simulink model "RM3_copy"  (R2017b)
settings: Solver=ode4  StartTime=0  StopTime=14400  FixedStep=0.1  MaxStep=0.1  RelTol=1e-3  EnableMultiTasking=on
values from neighbouring files (symbols this model uses):
  m = min(Out,[],2)    [ContinousControl.m]    (also in RL.m; RealTime_modif22.m)
  N = No*n    (= 60)    [ACTOR_CRITIC & SARSA.m]    (also in TDlearningExampleEforPosting.m)
  s = tf('s')    [Fe_extract.m]    (also in InputDataExtraction.m; LetsStartIt.m; SafeLetsStartIt.m; StateExtraction.m)
  states_space = states_spaceP    [ContinousControl.m]    (also in Forward_step.m = states_spaceP([1:9 6*9+1:9*7 15*9+1:9*16 5*9+1:9*6],:); RealTime_modif22.m)
  X = YX(:,2:end)    [L2adaptivepredictor.m]
  Y = YX(:,1)    [L2adaptivepredictor.m]
undefined symbols (not defined in the file or in its folder): body, constraint, pto, Z
libraries: nesl_utility x8, sm_lib x5, WECSim_Lib x4
settings Model: Creator=mlawson  LastModifiedBy=ghleila
settings SolverCC: ZeroCrossControl=DisableAll  AlgebraicLoopSolver=LineSearch  AutoInsertRateTranBlk=on
settings DataIOCC: SaveFormat=Array  SaveOutput=off  SaveTime=off
settings OptimizationCC: LifeSpan=inf  SimCompilerOptimization=on
settings DebuggingCC: UnderspecifiedInitializationDetection=Classic  MergeDetectMultiDrivingBlocksExec=none  SolverPrmCheckMsg=warning  AllowSymbolicDim=off  StateNameClashWarn=warning  SFUnexpectedBacktrackingDiag=warning  SFNoUnconditionalDefaultTransitionDiag=warning  SFExecutionAtInitializationDiag=none
settings HardwareCC: ProdBitPerPointer=32  ProdBitPerSizeT=32  ProdBitPerPtrDiffT=32  ProdLargestAtomicFloat=None  ProdIntDivRoundTo=Undefined  ProdEndianess=Unspecified  ProdWordSize=32  ProdHWDeviceType=32-bit Generic
settings ModelReferenceCC: PropagateSignalLabelsOutOfModel=off
settings CodeAppCC: StateflowObjectComments=on
settings GRTTargetCC: TargetLangStandard=C89/C90 (ANSI)  GeneratePreprocessorConditionals=Disable all
settings ConfigComp: CovMetricSettings=dw  CovHtmlReporting=on  CovSaveCumulativeToWorkspaceVar=on  CovSaveSingleToWorkspaceVar=on  CovExternalEMLEnable=off  CovSFcnEnable=off
settings SimscapeCC: SimscapeNormalizeSystem=off
settings ConfigurationSet: Description=SimMechanics 2G
settings ExplorerConfigSet: InternalSimMechanicsExplorerSettings="<ExplorerConfiguration><canonicalview>default</canonicalview><TilePanel><TileInfo><Tiles Columns=\"1\" Count=\"1\" Rows=\"1\"><Column Left=\"2\" Weight=\"1\"/><Column Left=\"1335\"/><Row Top=\"2\" Weight=\"1\"/><Row Top=\"911\"/><Tile Height=\"1\" Width=\"1\" X=\"0\" Y=\"0\"/></Tiles></TileInfo><SceneInfo><SceneViewer><BGColor><R>0.60000002384185791</R><G>0.60000002384185791</G><B>0.60000002384185791</B></BGColor><Camera><Position><X>365.37645888990272</X><Y>-369.82486814446582</Y><Z>359.64809521743916</Z></Position><Center><X>-6.7351450971904585</X><Y>2.2867358426280204</Y><Z>-12.463508769654169</Z></Center><Up><X>-0.40824829046386307</X><Y>0.40824829046386307</Y><Z>0.81649658092772615</Z></Up><Left>-57.820127362122818</Left><Right>57.820127362122818</Right><Bottom>-38.308817187253304</Bottom><Top>38.308817187253304</Top></Camera></SceneViewer></SceneInfo></TilePanel></ExplorerConfiguration>"

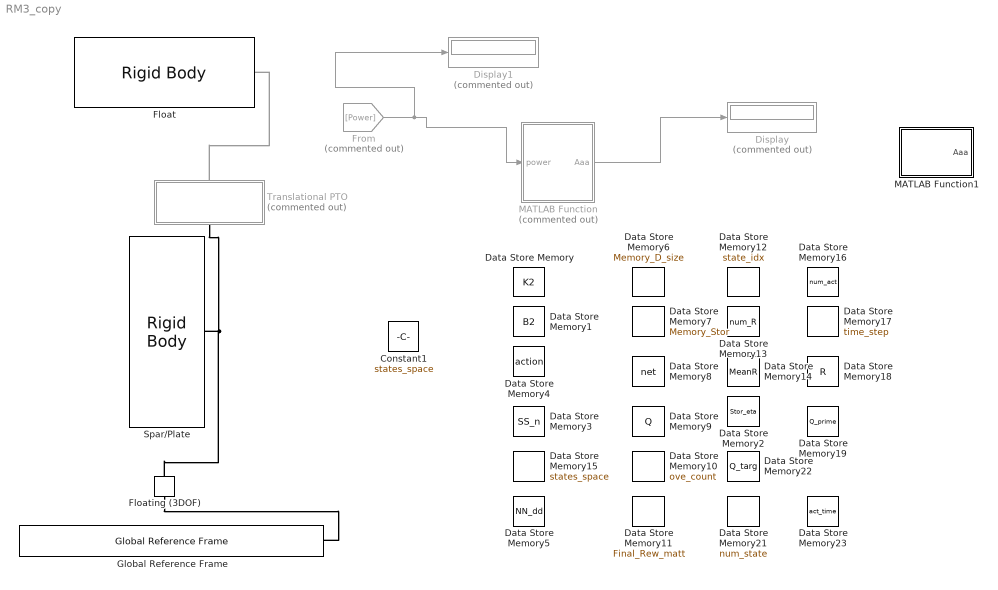
== system RM3_copy ==
  Constant1 : Constant  Value=states_space
  Data Store Memory : DataStoreMemory  DataStoreName=K2  ReadBeforeWriteMsg=warning  WriteAfterWriteMsg=warning  WriteAfterReadMsg=warning  InitialValue=K2  VectorParams1D=off  ShowAdditionalParam=off  OutDataTypeStr=double
  Data Store Memory1 : DataStoreMemory  DataStoreName=B2  ReadBeforeWriteMsg=warning  WriteAfterWriteMsg=warning  WriteAfterReadMsg=warning  InitialValue=B2  VectorParams1D=off  ShowAdditionalParam=off  OutDataTypeStr=double
  Data Store Memory10 : DataStoreMemory  DataStoreName=ove_count  ReadBeforeWriteMsg=warning  WriteAfterWriteMsg=warning  WriteAfterReadMsg=warning  InitialValue=1  VectorParams1D=off  ShowAdditionalParam=off  OutDataTypeStr=double
  Data Store Memory11 : DataStoreMemory  DataStoreName=Final_Rew_matt  ReadBeforeWriteMsg=warning  WriteAfterWriteMsg=warning  WriteAfterReadMsg=warning  ShowAdditionalParam=off  OutDataTypeStr=double
  Data Store Memory12 : DataStoreMemory  DataStoreName=state_idx  ReadBeforeWriteMsg=warning  WriteAfterWriteMsg=warning  WriteAfterReadMsg=warning  ShowAdditionalParam=off  OutDataTypeStr=int16
  Data Store Memory13 : DataStoreMemory  DataStoreName=num_R  ReadBeforeWriteMsg=warning  WriteAfterWriteMsg=warning  WriteAfterReadMsg=warning  VectorParams1D=off  ShowAdditionalParam=off  OutDataTypeStr=double
  Data Store Memory14 : DataStoreMemory  DataStoreName=MeanR  ReadBeforeWriteMsg=warning  WriteAfterWriteMsg=warning  WriteAfterReadMsg=warning  VectorParams1D=off  ShowAdditionalParam=off  OutDataTypeStr=double
  Data Store Memory15 : DataStoreMemory  DataStoreName=states_space  ReadBeforeWriteMsg=warning  WriteAfterWriteMsg=warning  WriteAfterReadMsg=warning  VectorParams1D=off  ShowAdditionalParam=off  OutDataTypeStr=double
  Data Store Memory16 : DataStoreMemory  DataStoreName=num_act  ReadBeforeWriteMsg=warning  WriteAfterWriteMsg=warning  WriteAfterReadMsg=warning  ShowAdditionalParam=off  OutDataTypeStr=double
  Data Store Memory17 : DataStoreMemory  DataStoreName=time_step  ReadBeforeWriteMsg=warning  WriteAfterWriteMsg=warning  WriteAfterReadMsg=warning  ShowAdditionalParam=off  OutDataTypeStr=double
  Data Store Memory18 : DataStoreMemory  DataStoreName=R  ReadBeforeWriteMsg=warning  WriteAfterWriteMsg=warning  WriteAfterReadMsg=warning  VectorParams1D=off  ShowAdditionalParam=off  OutDataTypeStr=double
  Data Store Memory19 : DataStoreMemory  DataStoreName=Q_prime  ReadBeforeWriteMsg=warning  WriteAfterWriteMsg=warning  WriteAfterReadMsg=warning  VectorParams1D=off  ShowAdditionalParam=off  OutDataTypeStr=double
  Data Store Memory2 : DataStoreMemory  DataStoreName=Stor_eta  ReadBeforeWriteMsg=warning  WriteAfterWriteMsg=warning  WriteAfterReadMsg=warning  VectorParams1D=off  ShowAdditionalParam=off  OutDataTypeStr=double
  Data Store Memory21 : DataStoreMemory  DataStoreName=num_state  ReadBeforeWriteMsg=warning  WriteAfterWriteMsg=warning  WriteAfterReadMsg=warning  ShowAdditionalParam=off  OutDataTypeStr=double
  Data Store Memory22 : DataStoreMemory  DataStoreName=Q_targ  ReadBeforeWriteMsg=warning  WriteAfterWriteMsg=warning  WriteAfterReadMsg=warning  VectorParams1D=off  ShowAdditionalParam=off  OutDataTypeStr=double
  Data Store Memory23 : DataStoreMemory  DataStoreName=act_time  ReadBeforeWriteMsg=warning  WriteAfterWriteMsg=warning  WriteAfterReadMsg=warning  ShowAdditionalParam=off  OutDataTypeStr=double
  Data Store Memory3 : DataStoreMemory  DataStoreName=SS_n  ReadBeforeWriteMsg=warning  WriteAfterWriteMsg=warning  WriteAfterReadMsg=warning  VectorParams1D=off  ShowAdditionalParam=off  OutDataTypeStr=double
  Data Store Memory4 : DataStoreMemory  DataStoreName=action  ReadBeforeWriteMsg=warning  WriteAfterWriteMsg=warning  WriteAfterReadMsg=warning  InitialValue=action  ShowAdditionalParam=off  OutDataTypeStr=double
  Data Store Memory5 : DataStoreMemory  DataStoreName=NN_dd  ReadBeforeWriteMsg=warning  WriteAfterWriteMsg=warning  WriteAfterReadMsg=warning  ShowAdditionalParam=off  OutDataTypeStr=double
  Data Store Memory6 : DataStoreMemory  DataStoreName=Memory_D_size  ReadBeforeWriteMsg=warning  WriteAfterWriteMsg=warning  WriteAfterReadMsg=warning  VectorParams1D=off  ShowAdditionalParam=off  OutDataTypeStr=double
  Data Store Memory7 : DataStoreMemory  DataStoreName=Memory_Stor  ReadBeforeWriteMsg=warning  WriteAfterWriteMsg=warning  WriteAfterReadMsg=warning  VectorParams1D=off  ShowAdditionalParam=off  OutDataTypeStr=double
  Data Store Memory8 : DataStoreMemory  DataStoreName=net  ReadBeforeWriteMsg=warning  WriteAfterWriteMsg=warning  WriteAfterReadMsg=warning  VectorParams1D=off  ShowAdditionalParam=off  OutDataTypeStr=double
  Data Store Memory9 : DataStoreMemory  DataStoreName=Q  ReadBeforeWriteMsg=warning  WriteAfterWriteMsg=warning  WriteAfterReadMsg=warning  VectorParams1D=off  ShowAdditionalParam=off  OutDataTypeStr=double
  Display : Display  Commented=on
  Display1 : Display  Commented=on
  Float : WECSim_Lib/Body Elements/Rigid Body  body=body(1)
      settings: AttributesFormatString=%<body>
  Floating (3DOF) : WECSim_Lib/Constraints/Floating (3DOF)  constraint=constraint(1)
      settings: AttributesFormatString=%<constraint>
  From : From  Commented=on  GotoTag=Power
  Global Reference Frame : WECSim_Lib/Frames/Global Reference Frame  waves=waves  simu=simu
  MATLAB Function : MATLAB Function  Commented=on  TreatAsAtomicUnit=on
  MATLAB Function1 : MATLAB Function  TreatAsAtomicUnit=on
  Spar/Plate : WECSim_Lib/Body Elements/Rigid Body  body=body(2)
      settings: AttributesFormatString=%<body>
  Translational PTO : Subsystem  Commented=on  AncestorBlock=WECSim_Lib/PTOs/Translational PTO  mask(PTO){pto=pto(1)}
      mask prompts: pto "PTO Name:"
      mask help:
      | Constraints the follower to translational motion relative to the base, in
      | the PTO's Z-direction and adds PTO stiffness and damping.
      |
      |
      | The variable name input below must be 'pto(i)' where i=1,2,...
      | pto(i) must be defined in the input file with the following fields:
      |
      |     .name (required)
      |             String.
      |             PTO name. Must comply with Matlab's variable naming rules.
      |     .loc (optional)
      |             3x1 vector [x y z] in meters.
      |             PTO location. Default = [0 0 0]
      |     .k (optional)
      |             Float.
      |             PTO linear spring stiffness. Default = 0
      |     .c (optional)
      |             Float.
      |             PTO linear damping coefficient. Default = 0
      |     .orientation.z (optional)
      |             3x1 vector [x y z].
      |             Direction of the PTO's Z-coordinate. Default = [0 0 1]
      |     .orientation.y (optional)
      |             3x1 vector [x y z].
      |             Direction of the PTO's Y-coordinate. Default = [0 1 0]
      mask init:
      | if exist('pto','var')
      |     h=[gcb '/output'];
      |     responseName=['pto' num2str(pto.ptoNum) '_out'];
      |     set_param(h,'VariableName',responseName);
      | end
      | 
      | pto.checkLoc('W');
      settings: AttributesFormatString=%<pto>
      mask Help:
      | Constraints the follower to translational motion relative to the base, in
      | the PTO's Z-direction and adds PTO stiffness and damping.
      | 
      | 
      | The variable name input below must be 'pto(i)' where i=1,2,...
      | pto(i) must be defined in the input file with the following fields:
      | 
      |     .name (required)
      |             String.
      |             PTO name. Must comply with Matlab's variable naming rules.
      |     .loc (optional)
      |             3x1 vector [x y z] in meters.
      |             PTO location. Default = [0 0 0]
      |     .k (optional)
      |             Float.
      |             PTO linear spring stiffness. Default = 0
      |     .c (optional)
      |             Float.
      |             PTO linear damping coefficient. Default = 0
      |     .orientation.z (optional)
      |             3x1 vector [x y z].
      |             Direction of the PTO's Z-coordinate. Default = [0 0 1]
      |     .orientation.y (optional)
      |             3x1 vector [x y z].
      |             Direction of the PTO's Y-coordinate. Default = [0 1 0]
  wires:
  From/1 -> MATLAB Function/1(power), Display1/1
  MATLAB Function/1(Aaa) -> Display/1
  connections:
  Floating (3DOF)/LConn1 -- Global Reference Frame/RConn1
  Spar/Plate/RConn1 -- Floating (3DOF)/RConn1 -- Translational PTO/RConn1
  Translational PTO/LConn1 -- Float/RConn1

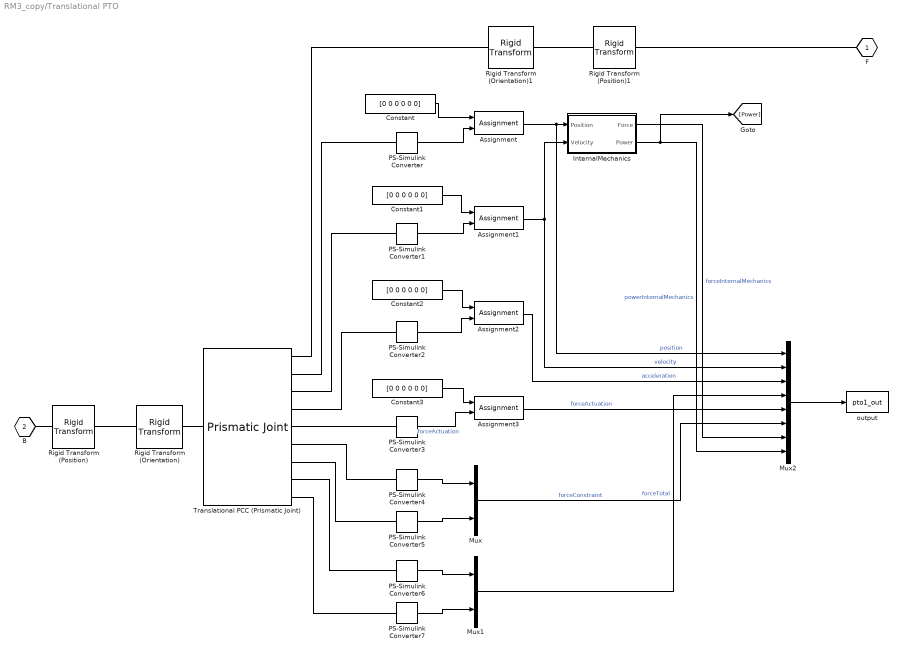
== system RM3_copy/Translational PTO ==
  Assignment{,1..3} (4 alike) : Assignment  IndexOptions=Index vector (dialog)  Indices=3  OutputSizes=1
  Constant{,1..3} (4 alike) : Constant  Value=[0 0 0 0 0 0]
  InternalMechanics : Subsystem
  Mux : Mux  Inputs=2
  Mux1 : Mux  Inputs=2
  Mux2 : Mux  Inputs=8
  PS-Simulink Converter{,1..7} (8 alike) : nesl_utility/PS-Simulink Converter  PhysicalDomain=network_engine_domain  SubClassName=ps_output  LeftPortType=input  RightPortType=output  PseudoPeriodic=off  Frequencies=[]  Unit=1  AffineConversion=off
  Rigid Transform (Position) : sm_lib/Frames and Transforms/Rigid Transform  TranslationMethod=Cartesian  TranslationStandardOffset=0  TranslationLengthUnit=m  TranslationStandardAxis=+Z  TranslationCartesianOffset=pto.initDisp.initLinDisp + pto.loc  TranslationROffset=0  TranslationROffsetUnits=m  TranslationZOffset=0  TranslationZOffsetUnits=m  TranslationThetaOffset=0  TranslationThetaOffsetUnits=deg  RotationMethod=None  RotationAngleUnits=rad  RotationStandardAxis=+Y  RotationAngle=0  RotationArbitraryAxis=[0 1 0]  FollAlignAxisA=+X  BaseAlignAxisA=+Y  FollAlignAxisB=+Y  BaseAlignAxisB=+Z  RotationSequenceAxes=FollowerAxes  RotationSequence=XYX  RotationSequenceAngles=[0 0 0]  RotationSequenceAnglesUnits=deg  RotationMatrix=[1 0 0; 0 1 0; 0 0 1]
  Rigid Transform (Position)1 : sm_lib/Frames and Transforms/Rigid Transform  TranslationMethod=Cartesian  TranslationStandardOffset=0  TranslationLengthUnit=m  TranslationStandardAxis=+Z  TranslationCartesianOffset=pto.initDisp.initLinDisp + pto.loc  TranslationROffset=0  TranslationROffsetUnits=m  TranslationZOffset=0  TranslationZOffsetUnits=m  TranslationThetaOffset=0  TranslationThetaOffsetUnits=deg  RotationMethod=None  RotationAngleUnits=rad  RotationStandardAxis=+Y  RotationAngle=0  RotationArbitraryAxis=[0 1 0]  FollAlignAxisA=+X  BaseAlignAxisA=+Y  FollAlignAxisB=+Y  BaseAlignAxisB=+Z  RotationSequenceAxes=FollowerAxes  RotationSequence=XYX  RotationSequenceAngles=[0 0 0]  RotationSequenceAnglesUnits=deg  RotationMatrix=[1 0 0; 0 1 0; 0 0 1]
  Rigid Transform (Orientation) : sm_lib/Frames and Transforms/Rigid Transform  TranslationMethod=None  TranslationStandardOffset=0  TranslationLengthUnit=m  TranslationStandardAxis=+Z  TranslationCartesianOffset=0  TranslationROffset=0  TranslationROffsetUnits=m  TranslationZOffset=0  TranslationZOffsetUnits=m  TranslationThetaOffset=0  TranslationThetaOffsetUnits=deg  RotationMethod=RotationMatrix  RotationAngleUnits=rad  RotationStandardAxis=+Y  RotationAngle=0  RotationArbitraryAxis=[0 1 0]  FollAlignAxisA=+X  BaseAlignAxisA=+Y  FollAlignAxisB=+Y  BaseAlignAxisB=+Z  RotationSequenceAxes=FollowerAxes  RotationSequence=XYX  RotationSequenceAngles=[0 0 0]  RotationSequenceAnglesUnits=deg  RotationMatrix=pto.orientation.rotationMatrix
  Rigid Transform (Orientation)1 : sm_lib/Frames and Transforms/Rigid Transform  TranslationMethod=None  TranslationStandardOffset=0  TranslationLengthUnit=m  TranslationStandardAxis=+Z  TranslationCartesianOffset=0  TranslationROffset=0  TranslationROffsetUnits=m  TranslationZOffset=0  TranslationZOffsetUnits=m  TranslationThetaOffset=0  TranslationThetaOffsetUnits=deg  RotationMethod=RotationMatrix  RotationAngleUnits=rad  RotationStandardAxis=+Y  RotationAngle=0  RotationArbitraryAxis=[0 1 0]  FollAlignAxisA=+X  BaseAlignAxisA=+Y  FollAlignAxisB=+Y  BaseAlignAxisB=+Z  RotationSequenceAxes=FollowerAxes  RotationSequence=XYX  RotationSequenceAngles=[0 0 0]  RotationSequenceAnglesUnits=deg  RotationMatrix=pto.orientation.rotationMatrix
  Translational PCC (Prismatic Joint) : sm_lib/Joints/Prismatic Joint  SenseConstraintForce=on  SenseConstraintForceX=off  SenseConstraintForceY=off  SenseConstraintForceZ=off  SenseConstraintTorque=on  SenseConstraintTorqueX=off  SenseConstraintTorqueY=off  SenseConstraintTorqueZ=off  SenseTotalForce=on  SenseTotalForceX=off  SenseTotalForceY=off  SenseTotalForceZ=off  SenseTotalTorque=on  SenseTotalTorqueX=off  SenseTotalTorqueY=off  SenseTotalTorqueZ=off  CompositeWrenchDir=BaseOnFollower  CompositeWrenchFrame=BaseFrame  EquilibriumPosition=0  EquilibriumPositionUnits=m  SpringStiffness=pto.k  SpringStiffnessUnits=N/m  DampingCoefficient=pto.c  DampingCoefficientUnits=N/(m/s)  TorqueActuationMode=NoTorque  MotionActuationMode=ComputedMotion  SensePosition=on  SenseVelocity=on  SenseAcceleration=on  SenseTorqueForce=on  PositionTargetSpecify=off  PositionTargetPriority=High  PositionTargetValue=0  PositionTargetValueUnits=m  VelocityTargetSpecify=off  VelocityTargetPriority=High  VelocityTargetValue=0  VelocityTargetValueUnits=m/s
  output : ToWorkspace  VariableName=pto1_out  SaveFormat=Structure With Time  SampleTime=-1
      settings: Decimation=round(simu.dtOut/simu.dt,0)
  F : PMIOPort  Port=1  Side=Left
  B : PMIOPort  Port=2  Side=Right
  wires:
  PS-Simulink Converter3/1 -> Assignment3/2  "forceActuation"
  Constant3/1 -> Assignment3/1
  InternalMechanics/2(Power) -> [Power], Mux2/8  "powerInternalMechanics"
  InternalMechanics/1(Force) -> Mux2/7  "forceInternalMechanics"
  PS-Simulink Converter2/1 -> Assignment2/2
  Constant2/1 -> Assignment2/1
  PS-Simulink Converter1/1 -> Assignment1/2
  Constant1/1 -> Assignment1/1
  PS-Simulink Converter/1 -> Assignment/2
  Constant/1 -> Assignment/1
  Assignment2/1 -> Mux2/3  "acceleration"
  Assignment1/1 -> InternalMechanics/2(Velocity), Mux2/2  "velocity"
  Assignment/1 -> InternalMechanics/1(Position), Mux2/1  "position"
  Assignment3/1 -> Mux2/5  "forceActuation"
  PS-Simulink Converter7/1 -> Mux1/2
  PS-Simulink Converter6/1 -> Mux1/1
  PS-Simulink Converter5/1 -> Mux/2
  PS-Simulink Converter4/1 -> Mux/1
  Mux1/1 -> Mux2/4  "forceTotal"
  Mux/1 -> Mux2/6  "forceConstraint"
  Mux2/1 -> output/1
  connections:
  Rigid Transform (Position)/RConn1 -- Rigid Transform (Orientation)/LConn1
  Rigid Transform (Position)1/RConn1 -- Rigid Transform (Orientation)1/LConn1
  Rigid Transform (Orientation)/RConn1 -- Translational PCC (Prismatic Joint)/LConn1
  Translational PCC (Prismatic Joint)/RConn6 -- PS-Simulink Converter4/LConn1
  Translational PCC (Prismatic Joint)/RConn2 -- PS-Simulink Converter/LConn1
  Translational PCC (Prismatic Joint)/RConn8 -- PS-Simulink Converter6/LConn1
  Rigid Transform (Position)1/LConn1 -- F/RConn1
  Translational PCC (Prismatic Joint)/RConn3 -- PS-Simulink Converter1/LConn1
  Translational PCC (Prismatic Joint)/RConn7 -- PS-Simulink Converter5/LConn1
  Translational PCC (Prismatic Joint)/RConn4 -- PS-Simulink Converter2/LConn1
  Rigid Transform (Orientation)1/RConn1 -- Translational PCC (Prismatic Joint)/RConn1
  Translational PCC (Prismatic Joint)/RConn9 -- PS-Simulink Converter7/LConn1
  Translational PCC (Prismatic Joint)/RConn5 -- PS-Simulink Converter3/LConn1
  Rigid Transform (Position)/LConn1 -- B/RConn1

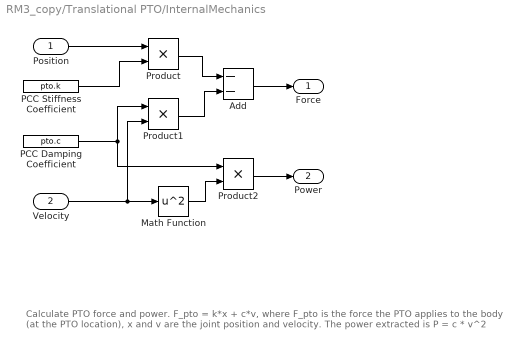
== system RM3_copy/Translational PTO/InternalMechanics ==
  note: Calculate PTO force and power.
      |
      | F_pto  = k*x + c*v,
      | where F_pto is the force the PTO applies to the body (at the PTO location), x and v are the joint position and velocity.
      |
      | The power extracted is
      | P = c * v^2
  Position : Inport
  Velocity : Inport  Port=2
  Add : Sum  Inputs=--
  Math Function : Math  Operator=square  SaturateOnIntegerOverflow=on
  PCC Damping Coefficient : Constant  Value=pto.c
  PCC Stiffness Coefficient : Constant  Value=pto.k
  Product : Product  Inputs=**
  Product1 : Product  Inputs=**
  Product2 : Product  Inputs=**
  Force : Outport
  Power : Outport  Port=2
  wires:
  Product1/1 -> Add/2
  Product/1 -> Add/1
  Math Function/1 -> Product2/2
  Add/1 -> Force/1
  Position/1 -> Product/1
  PCC Stiffness Coefficient/1 -> Product/2
  Velocity/1 -> Product1/2, Math Function/1
  Product2/1 -> Power/1
  PCC Damping Coefficient/1 -> Product1/1, Product2/1

== matlab function RM3_copy/MATLAB Function1 ==
  data: Aaa output; ove_count data_store_memory; action data_store_memory
function Aaa=fcn1

global ove_count action 
% B2 K2 act_time  SS_n  NN_dd Memory_D_size Memory_Stor  Q ...
%       state_idx  states_space  Stor_eta num_R MeanR  Q_targ num_state num_act time_step Q_prime  R Final_Rew_matt;


Aaa=1;

power=50;






%  pow=power(end-act_time/time_step:end);
% 
% mean_six_pow=mean(pow);
% PptoAvg=mean_six_pow;





%% initial state
    
   % for ove_count1=1:1500
  
        coder.extrinsic('num2str','datasample','get_param','feedforwardnet'); 
        
        
   
        disp(['iteration: ' num2str(ove_count)]);
        
        %     if ove_count>=500
        %
        %          gamma=gamma_int/((ove_count)^-0.06);
        %     else
        %
        %         gamma=gamma_int;
        %
        %     end
         
        if ove_count>=400
            
            gamma=0.6;
            opts.StepRatio = 0.01;
        else
            
            gamma=0.4;
            opts.StepRatio = 0.1;
            
        end
        
        
        
        if ove_count>=200
            
            alpha=0.6;
            
        else
            
            alpha=0.4;
            
        end
        
        
        
        %% Q value of the state usning NN
        
        %     if  ove_count> NN_dd+1
        %
        %       %  Q(state_idx,:) = v2h(dnn,states_space(state_idx,:));   % update q values
        %
        %       y = net(states_space(state_idx,:)');   % update q values
        %
        %       Q(state_idx,:)=y';
        %
        %     end
        
        
       %%% epsilon=epsilon_int;
        
        %% taking an action
        
        % % % % %     r=rand; % get 1 uniform random number
        % % % % %
        % % % % %     x=sum(r>=cumsum([0, 1-epsilon, epsilon])) % check it to be in which probability area
        % % % % %     % choose either explore or exploit
        % % % % %
        % % % % %     if x == 1   % exploit
        % % % % %
        % % % % %         [~,umax]=max(Q(state_idx,:));
        % % % % %
        % % % % %         % [~,umax]=max(V(state_idx,1));
        % % % % %
        % % % % %         current_action = action(umax,:);
        % % % % %
        % % % % %     else        % explore
        
        
       % coder.extrinsic('get_param');
  
       current_action=zeros(1,2); 
        
        [current_action]=datasample(action,1); % choose 1 action randomly (uniform random distribution)

== matlab function RM3_copy/MATLAB Function ==
  data: Memory_Stor data_store_memory; Q data_store_memory; ove_count data_store_memory; num_R data_store_memory; MeanR data_store_memory; Q_targ data_store_memory; Q_prime data_store_memory; R data_store_memory; K2 data_store_memory; act_time data_store_memory; SS_n data_store_memory; NN_dd data_store_memory; Memory_D_size data_store_memory; num_state data_store_memory; num_act data_store_memory; time_step data_store_memory; Aaa output double; B2 data_store_memory; power input; Final_Rew_matt data_store_memory; state_idx data_store_memory; Stor_eta data_store_memory; action data_store_memory; states_space data_store_memory
function Aaa=fcn1( power)

global B2 K2 act_time  SS_n  NN_dd Memory_D_size Memory_Stor  Q ove_count...
      state_idx  states_space action Stor_eta num_R MeanR  Q_targ num_state num_act time_step Q_prime  R Final_Rew_matt;


Aaa=1;








%  pow=power(end-act_time/time_step:end);
% 
% mean_six_pow=mean(pow);
% PptoAvg=mean_six_pow;





%% initial state
    
   % for ove_count1=1:1500
  
        coder.extrinsic('num2str','datasample','get_param','feedforwardnet'); 
        
        
   
        disp(['iteration: ' num2str(ove_count)]);
        
        %     if ove_count>=500
        %
        %          gamma=gamma_int/((ove_count)^-0.06);
        %     else
        %
        %         gamma=gamma_int;
        %
        %     end
         
        if ove_count>=400
            
            gamma=0.6;
            opts.StepRatio = 0.01;
        else
            
            gamma=0.4;
            opts.StepRatio = 0.1;
            
        end
        
        
        
        if ove_count>=200
            
            alpha=0.6;
            
        else
            
            alpha=0.4;
            
        end
        
        
        
        %% Q value of the state usning NN
        
        %     if  ove_count> NN_dd+1
        %
        %       %  Q(state_idx,:) = v2h(dnn,states_space(state_idx,:));   % update q values
        %
        %       y = net(states_space(state_idx,:)');   % update q values
        %
        %       Q(state_idx,:)=y';
        %
        %     end
        
        
       %%% epsilon=epsilon_int;
        
        %% taking an action
        
        % % % % %     r=rand; % get 1 uniform random number
        % % % % %
        % % % % %     x=sum(r>=cumsum([0, 1-epsilon, epsilon])) % check it to be in which probability area
        % % % % %     % choose either explore or exploit
        % % % % %
        % % % % %     if x == 1   % exploit
        % % % % %
        % % % % %         [~,umax]=max(Q(state_idx,:));
        % % % % %
        % % % % %         % [~,umax]=max(V(state_idx,1));
        % % % % %
        % % % % %         current_action = action(umax,:);
        % % % % %
        % % % % %     else        % explore
        
        
       % coder.extrinsic('get_param');
     
       current_action1=zeros(1,2); 
      
     action1=[3 4;4 5;4 7]
      % action_idx=zeros(1,1); 
        
        [current_action1]=datasample(action1,1); % choose 1 action randomly (uniform random distribution)
        
     %  action_idx = find(action(:,1)==current_action(1,1) & action(:,2)==current_action(1,2)); % id of the chosen action
%         


%        b=action(action_idx,1); %% DAMPING N/(m/s)
%        B2=b(1,1);
%        
%      
%        
% % %         
% % % %        %B2=max(B2Matrix);
%        k=action(action_idx,2);
%        K2=k(1,1);
%        
%          
% %         
%         %% storing eta for reconstruction 
% %         
%        
% Stor_eta(ove_count,1)=state_idx;
% %         %Stor_eta(ove_count,2)=irreg_eta_idx
% 
% [d f]=size(int(action_idx))
%         
      % Stor_eta(ove_count,2)=action_idx;
% %         
%         %% produce eta for the current state
%         
% % %         tsim_ove=60*Ts;  %%
% % %         delta_t=0.01;
% % %         StepT_SIM=0.01;
%         
%         %% next_state
%         
%         Height =states_space( state_idx,1);           %m         %Amplitude of the waves
%         
%         Ts =states_space( state_idx,2);
%         
%         
%         
%         next_stPrimee_idx=find(states_space(:,1)==Height & states_space(:,2)==Ts & states_space(:,3)==B2 & states_space(:,4)==K2);
% 
% % %         FeWithTime=[];
% % %         
% % %         FeWithTime=makeEtaFe(Height,Ts,tsim_ove,delta_t,A1,B1,K1);
% % %         
% % %         [PptoAvg]=TstSimulatorF(FeWithTime,A1,B1,K1,B2,K2,tsim_ove,StepT_SIM,state_idx);   % initiaL STATE
% % %       
% % %         wecSimInputFile;
% % %         wecSim;
% % %        %%% userDefinedFunctions
% % %         PP=output.ptos.powerInternalMechanics;
% % %         
% % %         mean_six_pow=mean(PP);
% % %         PptoAvg=mean_six_pow(1,3)
% % %         
% % %         hg(ove_count1)=PptoAvg;
% 
%         %% next state
%         st_chosen=double(0); 
%         st_chosen=datasample(1:size(states_space,1),1); % choose 1 action randomly (uniform random distribution)
%         
%         
%         Height_prime =states_space( st_chosen,1);           %m         %Amplitude of the waves
%         Ts_prime =states_space( st_chosen,2);             %s         %Significant period of the Wave
%         
%         next_state_idx=find(states_space(:,1)==Height_prime & states_space(:,2)==Ts_prime & states_space(:,3)==B2 & states_space(:,4)==K2);
%         
%         
%         %% allocating power
%         num_R(next_stPrimee_idx)=num_R(next_stPrimee_idx)+1;
%         next_reward=(PptoAvg/(Height^2)); %% normalized reward
%         %num_R(state_idx)=2;
%         R(next_stPrimee_idx,num_R(next_stPrimee_idx))=next_reward;
%         Height=states_space(next_stPrimee_idx,1);
%         
%         next_state_idx;
%         
%         Period=states_space(next_stPrimee_idx,2);
%         
%         R_idx=find(states_space(:,1)==Height& states_space(:,2)==Period);
%         
%         MeanR(R_idx,1)=sum(R(R_idx,:),2)./num_R(R_idx); % mean
%         
%         % MaxR=max(max(R(R_idx)));
%         
%         MaxR=max(MeanR(R_idx));
%         
%         Final_Rew_matt(R_idx)=MeanR(R_idx,1)/MaxR;
%         
%         Final_Rew=Final_Rew_matt(next_stPrimee_idx);
%         
%         Final_Rew=(Final_Rew)^5;
%         
% % %         if (PptoAvg/1e06)<=0.1
% % %             Final_Rew=-1;
% % %         end
%         
%         %     if ove_count>150
%         %
%         %         if Final_Rew==1
%         %         Final_Rew=10;
%         %         end
%         %     end
%         
%        % Stor_eta(ove_count,3)=(All_params3(1,1)); Stor_eta(ove_count,4)=(All_params3(1,2)); 
%        %%% so what
%         Stor_eta(ove_count,3)=B2;
%         Stor_eta(ove_count,4)=K2;  Stor_eta(ove_count,5)=PptoAvg;
%         
%         %% storing features
%         
%        % All_features(ove_count,:)=All_params3;  %%% to get an idea about the max of each parameter
%         
%         disp(['current state : ' num2str(state_idx) ' next state : ' num2str(next_state_idx) ' taken action : ' num2str(action(action_idx,:))]);
%         
%         disp([' next reward : ' num2str(Final_Rew)]);
%         
%         %% neural network part
%         
%         if ove_count> NN_dd  %% start traing network
%             
%                         %% droping off very old data
%             
%             if ove_count>Memory_D_size %% dropoff
%                 
%                 In=Memory_Stor(end-Memory_D_size+1:end,5:8);
%                 
%                 Output=Memory_Stor(end-Memory_D_size+1:end,9:end);
%                 
%                 nodes = [size(In,2) size(action,1)];
%                 
%             else
%                 
%                 In=Memory_Stor(:,5:8);
%                 
%                 Output=Memory_Stor(:,9:end);
%                 
%                 nodes = [size(In,2) size(action,1)];
%                 
%             end
%             
%             
% % % % %             
% % % % %             In=Memory_Stor(:,5:8);
% % % % %             
% % % % %             Output=Memory_Stor(:,9:end);
% % % % %             
%             
%                 Out=[];
%                 Out=Output;
%                 m = min(Out,[],2);
%                 range = max(Out,[],2) - m;
%                 Out= (Out - m) ./ range;
%             
%                 Input=[];
%                 Input=In;
%                 m11 = min(Input);
%                 range = max(Input) - m11;
%                 Input = (Input - m11) ./ range;
%             
%             
%             net = feedforwardnet([5]);
%             [net,tr] = train(net,Input',Out');
% %             
% %             
%             y_prime= net(states_space(next_state_idx,:)');
%             Q_prime(next_state_idx,:) =y_prime';
%             
%             
%         
%             
%             
% %             % % % %
% % % dnn=[];
% % %                 [dnn,out_est,rmse]=DNNf(Input,Output,nodes,opts);
% % %             Input;
% % %                 g=v2h(dnn, SS_n(next_state_idx,:));
% % %             
% % %                Q_prime(next_state_idx,:) = v2h(dnn, SS_n(next_state_idx,:));
% %             
%             
%             Q_targ(state_idx,action_idx)=Final_Rew+gamma*max(Q_prime(next_state_idx,:)); % update q values
%             
%             target=Q;
%             Q_prev=Q;
%             
%             target(state_idx,action_idx)=Q_targ(state_idx,action_idx); %%% update target
%             Memory_Stor(ove_count,:)=[state_idx,action_idx,Final_Rew,next_state_idx,states_space(state_idx,:),target(state_idx,:)];
% 
%             %% training NN with recent data
%             %        [dnn,out_est,rmse]=DNNf(Input,Output,nodes,opts);
%             
% % % %             error(tt)=rmse;
% % % %             tt=tt+1;
%         else
%             % Q_prev=Q;
%             
%             Q(state_idx,action_idx)=Q(state_idx,action_idx)+alpha*(Final_Rew+gamma*max(Q(next_state_idx,:))-Q(state_idx,action_idx));
%             
%             target=Q;
%             
%             Memory_Stor(ove_count,:)=[state_idx,action_idx,Final_Rew,next_state_idx,states_space(state_idx,:),target(state_idx,:)];
%         end
%         
%         %% checking the convergence of  Q function
%         
%         Q=target;
%         
%         % dif(ove_count)=norm(target(:,:)-Q_prev(:,:),Inf);
%         
%         ove_count=ove_count+1;
%         
%         state_idx=next_state_idx;
%         
%    % end
%     
% 
% 
% k=1;
% 
% 
% 
% 
% % % % 
% % % % %  end
% % % % 
% % % % num=size(SS_n,1);
% % % % num2=num/12;
% % % % 
% % % % for j=1:num2
% % % % [kk(j) jj(j)]=max(MeanR(12*(j-1)+1:12*(j)));
% % % % end
% % % % 
% % % % 
% % % % 
% % % % save('finallll')
% % % % 
% % % % 
% % % % 
% % % % save('power & Features','All_features')
% 
% 
% 
% 
% ove_count=ove_count+1;
% 
% 
% end
% 
% 
% 
%
